simulink library "lib_env"  (Simulink 7.7)
settings: Solver=ode45  StartTime=0.0  StopTime=10.0  RelTol=1e-3
undefined symbols (not defined in the file): ADSW, area, arm, CD, CGP, CR, Earth, earth_radius, ele, GE, GGSW, GPperturbationSW, I, J2, jd, pSR, q_ini, rem_mag, rem_magSW, SGP, SRPSW, TOLERANCE, UT1_UTC, w_ini, wE, WGS84
libraries: lib_util x20, aerolibutil x13, lib_env x10, lib_orbittrance x9, aerolibtransform2 x6, lib_astrodynamics x5, aerolibatmos2 x1, vrlib x1, aerolibgravity2 x1
(part 2 of 2)

== matlab function IGRF11/IGRF11 ==
  data: fyears input double; B output double; alt input double; nlat input double; elong input double
function B=fnc(fyears,alt,nlat,elong)
%****************************************************
%  Direct conversion of igrf11_f to MATLAB
%  USAGE:   [B]=igrf11syn(fyears,alt,nlat,elong) 
% 
%  INPUT:   fyears = date in fractional years e.g. 1909.5 
%           alt    = altitude in                       (km)
%           nlat   = latiude positive north            (deg)
%           elong  = longitude positive east           (deg)
% OUTPUT:
%                B = [B_North; B_East; B_Up]           (nano Teslas)   ←間違い
%                B = [B_North; B_East; B_Down]         (nano Teslas)
% 2011/09/15 Update
% プログラムはNEDなのに、ここの表記がNEUになっていたのでNEDに変更
% この北極付近でプログラムの出力の第三成分は正の値になっていたことにより発覚
% (地磁気は北極がS極で、南極がN極なので北極付近では磁場ベクトルが地心方向を向く。
%  つまりDown方向を向く)
% ちなみにIGRF公式のc言語のプログラムにはNEDと書いてあった。

%  Conversion written by
%  Charles L. Rino
%  Rino Consulting
%  September 27 2010/October 3 2010 
%  crino@mindspring.com
%
%  CHANGES
%  date replaced by fyears
%  colat replaced by nlat
%  isv and itype preset to 0 and 1, respectively
%  output changed from [x,y,z,f] to non-redundant vector B=[x; y; z];
%The following text is from the fortran comment lines:
%
%     This is a program for synthesising geomagnetic field values from the 
%     International Geomagnetic Reference Field series of models as agreed
%     in December 2009 by IAGA Working Group V-MOD. 
%     It is the 11th generation IGRF, ie the 10th revision. 
%     The main-field models for 1900.0, 1905.0,..1940.0 and 2010.0 are 
%     non-definitive, those for 1945.0, 1950.0,...2005.0 are definitive and
%     the secular-variation model for 2010.0 to 2015.0 is non-definitive.
%
%     Main-field models are to degree and order 10 (ie 120 coefficients)
%     for 1900.0-1995.0 and to 13 (ie 195 coefficients) for 2000.0 onwards. 
%     The predictive secular-variation model is to degree and order 8 (ie 80
%     coefficients).
%
%     Options include values at different locations at different
%     times (spot), values at same location at one year intervals
%     (time series), grid of values at one time (grid); geodetic or
%     geocentric coordinates, latitude & longitude entered as decimal
%     degrees or degrees & minutes (not in grid), choice of main field 
%     or secular variation or both (grid only).
% Recent history of code:
%     Aug 2003: 
%     Adapted from 8th generation version to include new maximum degree for
%     main-field models for 2000.0 and onwards and use WGS84 spheroid instead
%     of International Astronomical Union 1966 spheroid as recommended by IAGA
%     in July 2003. Reference radius remains as 6371.2 km - it is NOT the mean
%     radius (= 6371.0 km) but 6371.2 km is what is used in determining the
%     coefficients. 
%     Dec 2004: 
%     Adapted for 10th generation
%     Jul 2005: 
%     1995.0 coefficients as published in igrf9coeffs.xls and igrf10coeffs.xls
%     now used in code - (Kimmo Korhonen spotted 1 nT difference in 11 coefficients)
%     Dec 2009:
%     Adapted for 11th generation
%
%   INPUT
%     isv   = 0 if main-field values are required
%     isv   = 1 if secular variation values are required
%     date  = year A.D. Must be greater than or equal to 1900.0 and
%             less than or equal to 2015.0. Warning message is given
%             for dates greater than 2010.0. Must be double precision.
%     itype = 1 if geodetic (spheroid)
%     itype = 2 if geocentric (sphere)
%     alt   = height in km above sea level if itype = 1
%           = distance from centre of Earth in km if itype = 2 (>3485 km)
%     colat = colatitude (0-180)
%     elong = east-longitude (0-360)
%     alt, colat and elong must be double precision.
%   OUTPUT
%     x     = north component (nT) if isv = 0, nT/year if isv = 1
%     y     = east component (nT) if isv = 0, nT/year if isv = 1
%     z     = vertical component (nT) if isv = 0, nT/year if isv = 1
%     f     = total intensity (nT) if isv = 0, rubbish if isv = 1
%     B     = [x; y; z]
%
%     To get the other geomagnetic elements (D, I, H and secular
%     variations dD, dH, dI and dF) use routines ptoc and ptocsv.
%
%     Adapted from 8th generation version to include new maximum degree for
%     main-field models for 2000.0 and onwards and use WGS84 spheroid instead
%     of International Astronomical Union 1966 spheroid as recommended by IAGA
%     in July 2003. Reference radius remains as 6371.2 km - it is NOT the mean
%     radius (= 6371.0 km) but 6371.2 km is what is used in determining the
%     coefficients. Adaptation by Susan Macmillan, August 2003 (for
%     9th generation) and December 2004.
%     1995.0 coefficients as published in igrf9coeffs.xls and igrf10coeffs.xls
%     used - (Kimmo Korhonen spotted 1 nT difference in 11 coefficients)
%     Susan Macmillan July 2005
%************************************************************************************
%global gh
gh = [-31543,-2298,5922,-677,2905,-1061,924,1121,1022,-1469,-330,1256,3,572,523,876,628,195,660,-69,-361,-210,134,-75,-184,328,-210,264,53,5,-33,-86,-124,-16,3,63,61,-9,-11,83,-217,2,-58,-35,59,36,-90,-69,70,-55,-45,0,-13,34,-10,-41,-1,-21,28,18,-12,6,-22,11,8,8,-4,-14,-9,7,1,-13,2,5,-9,16,5,-5,8,-18,8,10,-20,1,14,-11,5,12,-3,1,-2,-2,8,2,10,-1,-2,-1,2,-3,-4,2,2,1,-5,2,-2,6,6,-4,4,0,0,-2,2,4,2,0,0,-6,-31464,-2298,5909,-728,2928,-1086,1041,1065,1037,-1494,-357,1239,34,635,480,880,643,203,653,-77,-380,-201,146,-65,-192,328,-193,259,56,-1,-32,-93,-125,-26,11,62,60,-7,-11,86,-221,4,-57,-32,57,32,-92,-67,70,-54,-46,0,-14,33,-11,-41,0,-20,28,18,-12,6,-22,11,8,8,-4,-15,-9,7,1,-13,2,5,-8,16,5,-5,8,-18,8,10,-20,1,14,-11,5,12,-3,1,-2,-2,8,2,10,0,-2,-1,2,-3,-4,2,2,1,-5,2,-2,6,6,-4,4,0,0,-2,2,4,2,0,0,-6,-31354,-2297,5898,-769,2948,-1128,1176,1000,1058,-1524,-389,1223,62,705,425,884,660,211,644,-90,-400,-189,160,-55,-201,327,-172,253,57,-9,-33,-102,-126,-38,21,62,58,-5,-11,89,-224,5,-54,-29,54,28,-95,-65,71,-54,-47,1,-14,32,-12,-40,1,-19,28,18,-13,6,-22,11,8,8,-4,-15,-9,6,1,-13,2,5,-8,16,5,-5,8,-18,8,10,-20,1,14,-11,5,12,-3,1,-2,-2,8,2,10,0,-2,-1,2,-3,-4,2,2,1,-5,2,-2,6,6,-4,4,0,0,-2,2,4,2,0,0,-6,-31212,-2306,5875,-802,2956,-1191,1309,917,1084,-1559,-421,1212,84,778,360,887,678,218,631,-109,-416,-173,178,-51,-211,327,-148,245,58,-16,-34,-111,-126,-51,32,61,57,-2,-10,93,-228,8,-51,-26,49,23,-98,-62,72,-54,-48,2,-14,31,-12,-38,2,-18,28,19,-15,6,-22,11,8,8,-4,-15,-9,6,2,-13,3,5,-8,16,6,-5,8,-18,8,10,-20,1,14,-11,5,12,-3,1,-2,-2,8,2,10,0,-2,-1,2,-3,-4,2,2,1,-5,2,-2,6,6,-4,4,0,0,-2,1,4,2,0,0,-6,-31060,-2317,5845,-839,2959,-1259,1407,823,1111,-1600,-445,1205,103,839,293,889,695,220,616,-134,-424,-153,199,-57,-221,326,-122,236,58,-23,-38,-119,-125,-62,43,61,55,0,-10,96,-233,11,-46,-22,44,18,-101,-57,73,-54,-49,2,-14,29,-13,-37,4,-16,28,19,-16,6,-22,11,7,8,-3,-15,-9,6,2,-14,4,5,-7,17,6,-5,8,-19,8,10,-20,1,14,-11,5,12,-3,1,-2,-2,9,2,10,0,-2,-1,2,-3,-4,2,2,1,-5,2,-2,6,6,-4,4,0,0,-2,1,4,3,0,0,-6,-30926,-2318,5817,-893,2969,-1334,1471,728,1140,-1645,-462,1202,119,881,229,891,711,216,601,-163,-426,-130,217,-70,-230,326,-96,226,58,-28,-44,-125,-122,-69,51,61,54,3,-9,99,-238,14,-40,-18,39,13,-103,-52,73,-54,-50,3,-14,27,-14,-35,5,-14,29,19,-17,6,-21,11,7,8,-3,-15,-9,6,2,-14,4,5,-7,17,7,-5,8,-19,8,10,-20,1,14,-11,5,12,-3,1,-2,-2,9,2,10,0,-2,-1,2,-3,-4,2,2,1,-5,2,-2,6,6,-4,4,0,0,-2,1,4,3,0,0,-6,-30805,-2316,5808,-951,2980,-1424,1517,644,1172,-1692,-480,1205,133,907,166,896,727,205,584,-195,-422,-109,234,-90,-237,327,-72,218,60,-32,-53,-131,-118,-74,58,60,53,4,-9,102,-242,19,-32,-16,32,8,-104,-46,74,-54,-51,4,-15,25,-14,-34,6,-12,29,18,-18,6,-20,11,7,8,-3,-15,-9,5,2,-14,5,5,-6,18,8,-5,8,-19,8,10,-20,1,14,-12,5,12,-3,1,-2,-2,9,3,10,0,-2,-2,2,-3,-4,2,2,1,-5,2,-2,6,6,-4,4,0,0,-2,1,4,3,0,0,-6,-30715,-2306,5812,-1018,2984,-1520,1550,586,1206,-1740,-494,1215,146,918,101,903,744,188,565,-226,-415,-90,249,-114,-241,329,-51,211,64,-33,-64,-136,-115,-76,64,59,53,4,-8,104,-246,25,-25,-15,25,4,-106,-40,74,-53,-52,4,-17,23,-14,-33,7,-11,29,18,-19,6,-19,11,7,8,-3,-15,-9,5,1,-15,6,5,-6,18,8,-5,7,-19,8,10,-20,1,15,-12,5,11,-3,1,-3,-2,9,3,11,0,-2,-2,2,-3,-4,2,2,1,-5,2,-2,6,6,-4,4,0,0,-1,2,4,3,0,0,-6,-30654,-2292,5821,-1106,2981,-1614,1566,528,1240,-1790,-499,1232,163,916,43,914,762,169,550,-252,-405,-72,265,-141,-241,334,-33,208,71,-33,-75,-141,-113,-76,69,57,54,4,-7,105,-249,33,-18,-15,18,0,-107,-33,74,-53,-52,4,-18,20,-14,-31,7,-9,29,17,-20,5,-19,11,7,8,-3,-14,-10,5,1,-15,6,5,-5,19,9,-5,7,-19,8,10,-21,1,15,-12,5,11,-3,1,-3,-2,9,3,11,1,-2,-2,2,-3,-4,2,2,1,-5,2,-2,6,6,-4,4,0,0,-1,2,4,3,0,0,-6,-30594,-2285,5810,-1244,2990,-1702,1578,477,1282,-1834,-499,1255,186,913,-11,944,776,144,544,-276,-421,-55,304,-178,-253,346,-12,194,95,-20,-67,-142,-119,-82,82,59,57,6,6,100,-246,16,-25,-9,21,-16,-104,-39,70,-40,-45,0,-18,0,2,-29,6,-10,28,15,-17,29,-22,13,7,12,-8,-21,-5,-12,9,-7,7,2,-10,18,7,3,2,-11,5,-21,-27,1,17,-11,29,3,-9,16,4,-3,9,-4,6,-3,1,-4,8,-3,11,5,1,1,2,-20,-5,-1,-1,-6,8,6,-1,-4,-3,-2,5,0,-2,-2,-30554,-2250,5815,-1341,2998,-1810,1576,381,1297,-1889,-476,1274,206,896,-46,954,792,136,528,-278,-408,-37,303,-210,-240,349,3,211,103,-20,-87,-147,-122,-76,80,54,57,-1,4,99,-247,33,-16,-12,12,-12,-105,-30,65,-55,-35,2,-17,1,0,-40,10,-7,36,5,-18,19,-16,22,15,5,-4,-22,-1,0,11,-21,15,-8,-13,17,5,-4,-1,-17,3,-7,-24,-1,19,-25,12,10,2,5,2,-5,8,-2,8,3,-11,8,-7,-8,4,13,-1,-2,13,-10,-4,2,4,-3,12,6,3,-3,2,6,10,11,3,8,-30500,-2215,5820,-1440,3003,-1898,1581,291,1302,-1944,-462,1288,216,882,-83,958,796,133,510,-274,-397,-23,290,-230,-229,360,15,230,110,-23,-98,-152,-121,-69,78,47,57,-9,3,96,-247,48,-8,-16,7,-12,-107,-24,65,-56,-50,2,-24,10,-4,-32,8,-11,28,9,-20,18,-18,11,9,10,-6,-15,-14,5,6,-23,10,3,-7,23,6,-4,9,-13,4,9,-11,-4,12,-5,7,2,6,4,-2,1,10,2,7,2,-6,5,5,-3,-5,-4,-1,0,2,-8,-3,-2,7,-4,4,1,-2,-3,6,7,-2,-1,0,-3,-30421,-2169,5791,-1555,3002,-1967,1590,206,1302,-1992,-414,1289,224,878,-130,957,800,135,504,-278,-394,3,269,-255,-222,362,16,242,125,-26,-117,-156,-114,-63,81,46,58,-10,1,99,-237,60,-1,-20,-2,-11,-113,-17,67,-56,-55,5,-28,15,-6,-32,7,-7,23,17,-18,8,-17,15,6,11,-4,-14,-11,7,2,-18,10,4,-5,23,10,1,8,-20,4,6,-18,0,12,-9,2,1,0,4,-3,-1,9,-2,8,3,0,-1,5,1,-3,4,4,1,0,0,-1,2,4,-5,6,1,1,-1,-1,6,2,0,0,-7,-30334,-2119,5776,-1662,2997,-2016,1594,114,1297,-2038,-404,1292,240,856,-165,957,804,148,479,-269,-390,13,252,-269,-219,358,19,254,128,-31,-126,-157,-97,-62,81,45,61,-11,8,100,-228,68,4,-32,1,-8,-111,-7,75,-57,-61,4,-27,13,-2,-26,6,-6,26,13,-23,1,-12,13,5,7,-4,-12,-14,9,0,-16,8,4,-1,24,11,-3,4,-17,8,10,-22,2,15,-13,7,10,-4,-1,-5,-1,10,5,10,1,-4,-2,1,-2,-3,2,2,1,-5,2,-2,6,4,-4,4,0,0,-2,2,3,2,0,0,-6,-30220,-2068,5737,-1781,3000,-2047,1611,25,1287,-2091,-366,1278,251,838,-196,952,800,167,461,-266,-395,26,234,-279,-216,359,26,262,139,-42,-139,-160,-91,-56,83,43,64,-12,15,100,-212,72,2,-37,3,-6,-112,1,72,-57,-70,1,-27,14,-4,-22,8,-2,23,13,-23,-2,-11,14,6,7,-2,-15,-13,6,-3,-17,5,6,0,21,11,-6,3,-16,8,10,-21,2,16,-12,6,10,-4,-1,-5,0,10,3,11,1,-2,-1,1,-3,-3,1,2,1,-5,3,-1,4,6,-4,4,0,1,-1,0,3,3,1,-1,-4,-30100,-2013,5675,-1902,3010,-2067,1632,-68,1276,-2144,-333,1260,262,830,-223,946,791,191,438,-265,-405,39,216,-288,-218,356,31,264,148,-59,-152,-159,-83,-49,88,45,66,-13,28,99,-198,75,1,-41,6,-4,-111,11,71,-56,-77,1,-26,16,-5,-14,10,0,22,12,-23,-5,-12,14,6,6,-1,-16,-12,4,-8,-19,4,6,0,18,10,-10,1,-17,7,10,-21,2,16,-12,7,10,-4,-1,-5,-1,10,4,11,1,-3,-2,1,-3,-3,1,2,1,-5,3,-2,4,5,-4,4,-1,1,-1,0,3,3,1,-1,-5,-29992,-1956,5604,-1997,3027,-2129,1663,-200,1281,-2180,-336,1251,271,833,-252,938,782,212,398,-257,-419,53,199,-297,-218,357,46,261,150,-74,-151,-162,-78,-48,92,48,66,-15,42,93,-192,71,4,-43,14,-2,-108,17,72,-59,-82,2,-27,21,-5,-12,16,1,18,11,-23,-2,-10,18,6,7,0,-18,-11,4,-7,-22,4,9,3,16,6,-13,-1,-15,5,10,-21,1,16,-12,9,9,-5,-3,-6,-1,9,7,10,2,-6,-5,2,-4,-4,1,2,0,-5,3,-2,6,5,-4,3,0,1,-1,2,4,3,0,0,-6,-29873,-1905,5500,-2072,3044,-2197,1687,-306,1296,-2208,-310,1247,284,829,-297,936,780,232,361,-249,-424,69,170,-297,-214,355,47,253,150,-93,-154,-164,-75,-46,95,53,65,-16,51,88,-185,69,4,-48,16,-1,-102,21,74,-62,-83,3,-27,24,-2,-6,20,4,17,10,-23,0,-7,21,6,8,0,-19,-11,5,-9,-23,4,11,4,14,4,-15,-4,-11,5,10,-21,1,15,-12,9,9,-6,-3,-6,-1,9,7,9,1,-7,-5,2,-4,-4,1,3,0,-5,3,-2,6,5,-4,3,0,1,-1,2,4,3,0,0,-6,-29775,-1848,5406,-2131,3059,-2279,1686,-373,1314,-2239,-284,1248,293,802,-352,939,780,247,325,-240,-423,84,141,-299,-214,353,46,245,154,-109,-153,-165,-69,-36,97,61,65,-16,59,82,-178,69,3,-52,18,1,-96,24,77,-64,-80,2,-26,26,0,-1,21,5,17,9,-23,0,-4,23,5,10,-1,-19,-10,6,-12,-22,3,12,4,12,2,-16,-6,-10,4,9,-20,1,15,-12,11,9,-7,-4,-7,-2,9,7,8,1,-7,-6,2,-3,-4,2,2,1,-5,3,-2,6,4,-4,3,0,1,-2,3,3,3,-1,0,-6,-29692,-1784,5306,-2200,3070,-2366,1681,-413,1335,-2267,-262,1249,302,759,-427,940,780,262,290,-236,-418,97,122,-306,-214,352,46,235,165,-118,-143,-166,-55,-17,107,68,67,-17,68,72,-170,67,-1,-58,19,1,-93,36,77,-72,-69,1,-25,28,4,5,24,4,17,8,-24,-2,-6,25,6,11,-6,-21,-9,8,-14,-23,9,15,6,11,-5,-16,-7,-4,4,9,-20,3,15,-10,12,8,-6,-8,-8,-1,8,10,5,-2,-8,-8,3,-3,-6,1,2,0,-4,4,-1,5,4,-5,2,-1,2,-2,5,1,1,-2,0,-7,0,0,0,0,0,0,0,0,0,0,0,0,0,0,0,0,0,0,0,0,0,0,0,0,0,0,0,0,0,0,0,0,0,0,0,0,0,0,0,0,0,0,0,0,0,0,0,0,0,0,0,0,0,0,0,0,0,0,0,0,0,0,0,0,0,0,0,0,0,0,0,0,0,0,0,-29619.4000000000,-1728.20000000000,5186.10000000000,-2267.70000000000,3068.40000000000,-2481.60000000000,1670.90000000000,-458,1339.60000000000,-2288,-227.600000000000,1252.10000000000,293.400000000000,714.500000000000,-491.100000000000,932.300000000000,786.800000000000,272.600000000000,250,-231.900000000000,-403,119.800000000000,111.300000000000,-303.800000000000,-218.800000000000,351.400000000000,43.8000000000000,222.300000000000,171.900000000000,-130.400000000000,-133.100000000000,-168.600000000000,-39.3000000000000,-12.9000000000000,106.300000000000,72.3000000000000,68.2000000000000,-17.4000000000000,74.2000000000000,63.7000000000000,-160.900000000000,65.1000000000000,-5.90000000000000,-61.2000000000000,16.9000000000000,0.700000000000000,-90.4000000000000,43.8000000000000,79,-74,-64.6000000000000,0,-24.2000000000000,33.3000000000000,6.20000000000000,9.10000000000000,24,6.90000000000000,14.8000000000000,7.30000000000000,-25.4000000000000,-1.20000000000000,-5.80000000000000,24.4000000000000,6.60000000000000,11.9000000000000,-9.20000000000000,-21.5000000000000,-7.90000000000000,8.50000000000000,-16.6000000000000,-21.5000000000000,9.10000000000000,15.5000000000000,7,8.90000000000000,-7.90000000000000,-14.9000000000000,-7,-2.10000000000000,5,9.40000000000000,-19.7000000000000,3,13.4000000000000,-8.40000000000000,12.5000000000000,6.30000000000000,-6.20000000000000,-8.90000000000000,-8.40000000000000,-1.50000000000000,8.40000000000000,9.30000000000000,3.80000000000000,-4.30000000000000,-8.20000000000000,-8.20000000000000,4.80000000000000,-2.60000000000000,-6,1.70000000000000,1.70000000000000,0,-3.10000000000000,4,-0.500000000000000,4.90000000000000,3.70000000000000,-5.90000000000000,1,-1.20000000000000,2,-2.90000000000000,4.20000000000000,0.200000000000000,0.300000000000000,-2.20000000000000,-1.10000000000000,-7.40000000000000,2.70000000000000,-1.70000000000000,0.100000000000000,-1.90000000000000,1.30000000000000,1.50000000000000,-0.900000000000000,-0.100000000000000,-2.60000000000000,0.100000000000000,0.900000000000000,-0.700000000000000,-0.700000000000000,0.700000000000000,-2.80000000000000,1.70000000000000,-0.900000000000000,0.100000000000000,-1.20000000000000,1.20000000000000,-1.90000000000000,4,-0.900000000000000,-2.20000000000000,-0.300000000000000,-0.400000000000000,0.200000000000000,0.300000000000000,0.900000000000000,2.50000000000000,-0.200000000000000,-2.60000000000000,0.900000000000000,0.700000000000000,-0.500000000000000,0.300000000000000,0.300000000000000,0,-0.300000000000000,0,-0.400000000000000,0.300000000000000,-0.100000000000000,-0.900000000000000,-0.200000000000000,-0.400000000000000,-0.400000000000000,0.800000000000000,-0.200000000000000,-0.900000000000000,-0.900000000000000,0.300000000000000,0.200000000000000,0.100000000000000,1.80000000000000,-0.400000000000000,-0.400000000000000,1.30000000000000,-1,-0.400000000000000,-0.100000000000000,0.700000000000000,0.700000000000000,-0.400000000000000,0.300000000000000,0.300000000000000,0.600000000000000,-0.100000000000000,0.300000000000000,0.400000000000000,-0.200000000000000,0,-0.500000000000000,0.100000000000000,-0.900000000000000,-29554.6300000000,-1669.05000000000,5077.99000000000,-2337.24000000000,3047.69000000000,-2594.50000000000,1657.76000000000,-515.430000000000,1336.30000000000,-2305.83000000000,-198.860000000000,1246.39000000000,269.720000000000,672.510000000000,-524.720000000000,920.550000000000,797.960000000000,282.070000000000,210.650000000000,-225.230000000000,-379.860000000000,145.150000000000,100,-305.360000000000,-227,354.410000000000,42.7200000000000,208.950000000000,180.250000000000,-136.540000000000,-123.450000000000,-168.050000000000,-19.5700000000000,-13.5500000000000,103.850000000000,73.6000000000000,69.5600000000000,-20.3300000000000,76.7400000000000,54.7500000000000,-151.340000000000,63.6300000000000,-14.5800000000000,-63.5300000000000,14.5800000000000,0.240000000000000,-86.3600000000000,50.9400000000000,79.8800000000000,-74.4600000000000,-61.1400000000000,-1.65000000000000,-22.5700000000000,38.7300000000000,6.82000000000000,12.3000000000000,25.3500000000000,9.37000000000000,10.9300000000000,5.42000000000000,-26.3200000000000,1.94000000000000,-4.64000000000000,24.8000000000000,7.62000000000000,11.2000000000000,-11.7300000000000,-20.8800000000000,-6.88000000000000,9.83000000000000,-18.1100000000000,-19.7100000000000,10.1700000000000,16.2200000000000,9.36000000000000,7.61000000000000,-11.2500000000000,-12.7600000000000,-4.87000000000000,-0.0600000000000000,5.58000000000000,9.76000000000000,-20.1100000000000,3.58000000000000,12.6900000000000,-6.94000000000000,12.6700000000000,5.01000000000000,-6.72000000000000,-10.7600000000000,-8.16000000000000,-1.25000000000000,8.10000000000000,8.76000000000000,2.92000000000000,-6.66000000000000,-7.73000000000000,-9.22000000000000,6.01000000000000,-2.17000000000000,-6.12000000000000,2.19000000000000,1.42000000000000,0.100000000000000,-2.35000000000000,4.46000000000000,-0.150000000000000,4.76000000000000,3.06000000000000,-6.58000000000000,0.290000000000000,-1.01000000000000,2.06000000000000,-3.47000000000000,3.77000000000000,-0.860000000000000,-0.210000000000000,-2.31000000000000,-2.09000000000000,-7.93000000000000,2.95000000000000,-1.60000000000000,0.260000000000000,-1.88000000000000,1.44000000000000,1.44000000000000,-0.770000000000000,-0.310000000000000,-2.27000000000000,0.290000000000000,0.900000000000000,-0.790000000000000,-0.580000000000000,0.530000000000000,-2.69000000000000,1.80000000000000,-1.08000000000000,0.160000000000000,-1.58000000000000,0.960000000000000,-1.90000000000000,3.99000000000000,-1.39000000000000,-2.15000000000000,-0.290000000000000,-0.550000000000000,0.210000000000000,0.230000000000000,0.890000000000000,2.38000000000000,-0.380000000000000,-2.63000000000000,0.960000000000000,0.610000000000000,-0.300000000000000,0.400000000000000,0.460000000000000,0.0100000000000000,-0.350000000000000,0.0200000000000000,-0.360000000000000,0.280000000000000,0.0800000000000000,-0.870000000000000,-0.490000000000000,-0.340000000000000,-0.0800000000000000,0.880000000000000,-0.160000000000000,-0.880000000000000,-0.760000000000000,0.300000000000000,0.330000000000000,0.280000000000000,1.72000000000000,-0.430000000000000,-0.540000000000000,1.18000000000000,-1.07000000000000,-0.370000000000000,-0.0400000000000000,0.750000000000000,0.630000000000000,-0.260000000000000,0.210000000000000,0.350000000000000,0.530000000000000,-0.0500000000000000,0.380000000000000,0.410000000000000,-0.220000000000000,-0.100000000000000,-0.570000000000000,-0.180000000000000,-0.820000000000000,-29496.5000000000,-1585.90000000000,4945.10000000000,-2396.60000000000,3026,-2707.70000000000,1668.60000000000,-575.400000000000,1339.70000000000,-2326.30000000000,-160.500000000000,1231.70000000000,251.700000000000,634.200000000000,-536.800000000000,912.600000000000,809,286.400000000000,166.600000000000,-211.200000000000,-357.100000000000,164.400000000000,89.7000000000000,-309.200000000000,-231.100000000000,357.200000000000,44.7000000000000,200.300000000000,188.900000000000,-141.200000000000,-118.100000000000,-163.100000000000,0.100000000000000,-7.70000000000000,100.900000000000,72.8000000000000,68.6000000000000,-20.8000000000000,76,44.2000000000000,-141.400000000000,61.5000000000000,-22.9000000000000,-66.3000000000000,13.1000000000000,3.10000000000000,-77.9000000000000,54.9000000000000,80.4000000000000,-75,-57.8000000000000,-4.70000000000000,-21.2000000000000,45.3000000000000,6.60000000000000,14,24.9000000000000,10.4000000000000,7,1.60000000000000,-27.7000000000000,4.90000000000000,-3.40000000000000,24.3000000000000,8.20000000000000,10.9000000000000,-14.5000000000000,-20,-5.70000000000000,11.9000000000000,-19.3000000000000,-17.4000000000000,11.6000000000000,16.7000000000000,10.9000000000000,7.10000000000000,-14.1000000000000,-10.8000000000000,-3.70000000000000,1.70000000000000,5.40000000000000,9.40000000000000,-20.5000000000000,3.40000000000000,11.6000000000000,-5.30000000000000,12.8000000000000,3.10000000000000,-7.20000000000000,-12.4000000000000,-7.40000000000000,-0.800000000000000,8,8.40000000000000,2.20000000000000,-8.40000000000000,-6.10000000000000,-10.1000000000000,7,-2,-6.30000000000000,2.80000000000000,0.900000000000000,-0.100000000000000,-1.10000000000000,4.70000000000000,-0.200000000000000,4.40000000000000,2.50000000000000,-7.20000000000000,-0.300000000000000,-1,2.20000000000000,-4,3.10000000000000,-2,-1,-2,-2.80000000000000,-8.30000000000000,3,-1.50000000000000,0.100000000000000,-2.10000000000000,1.70000000000000,1.60000000000000,-0.600000000000000,-0.500000000000000,-1.80000000000000,0.500000000000000,0.900000000000000,-0.800000000000000,-0.400000000000000,0.400000000000000,-2.50000000000000,1.80000000000000,-1.30000000000000,0.200000000000000,-2.10000000000000,0.800000000000000,-1.90000000000000,3.80000000000000,-1.80000000000000,-2.10000000000000,-0.200000000000000,-0.800000000000000,0.300000000000000,0.300000000000000,1,2.20000000000000,-0.700000000000000,-2.50000000000000,0.900000000000000,0.500000000000000,-0.100000000000000,0.600000000000000,0.500000000000000,0,-0.400000000000000,0.100000000000000,-0.400000000000000,0.300000000000000,0.200000000000000,-0.900000000000000,-0.800000000000000,-0.200000000000000,0,0.800000000000000,-0.200000000000000,-0.900000000000000,-0.800000000000000,0.300000000000000,0.300000000000000,0.400000000000000,1.70000000000000,-0.400000000000000,-0.600000000000000,1.10000000000000,-1.20000000000000,-0.300000000000000,-0.100000000000000,0.800000000000000,0.500000000000000,-0.200000000000000,0.100000000000000,0.400000000000000,0.500000000000000,0,0.400000000000000,0.400000000000000,-0.200000000000000,-0.300000000000000,-0.500000000000000,-0.300000000000000,-0.800000000000000,11.4000000000000,16.7000000000000,-28.8000000000000,-11.3000000000000,-3.90000000000000,-23,2.70000000000000,-12.9000000000000,1.30000000000000,-3.90000000000000,8.60000000000000,-2.90000000000000,-2.90000000000000,-8.10000000000000,-2.10000000000000,-1.40000000000000,2,0.400000000000000,-8.90000000000000,3.20000000000000,4.40000000000000,3.60000000000000,-2.30000000000000,-0.800000000000000,-0.500000000000000,0.500000000000000,0.500000000000000,-1.50000000000000,1.50000000000000,-0.700000000000000,0.900000000000000,1.30000000000000,3.70000000000000,1.40000000000000,-0.600000000000000,-0.300000000000000,-0.300000000000000,-0.100000000000000,-0.300000000000000,-2.10000000000000,1.90000000000000,-0.400000000000000,-1.60000000000000,-0.500000000000000,-0.200000000000000,0.800000000000000,1.80000000000000,0.500000000000000,0.200000000000000,-0.100000000000000,0.600000000000000,-0.600000000000000,0.300000000000000,1.40000000000000,-0.200000000000000,0.300000000000000,-0.100000000000000,0.100000000000000,-0.800000000000000,-0.800000000000000,-0.300000000000000,0.400000000000000,0.200000000000000,-0.100000000000000,0.100000000000000,0,-0.500000000000000,0.200000000000000,0.300000000000000,0.500000000000000,-0.300000000000000,0.400000000000000,0.300000000000000,0.100000000000000,0.200000000000000,-0.100000000000000,-0.500000000000000,0.400000000000000,0.200000000000000,0.400000000000000,0,0,0,0,0,0,0,0,0,0,0,0,0,0,0,0,0,0,0,0,0,0,0,0,0,0,0,0,0,0,0,0,0,0,0,0,0,0,0,0,0,0,0,0,0,0,0,0,0,0,0,0,0,0,0,0,0,0,0,0,0,0,0,0,0,0,0,0,0,0,0,0,0,0,0,0,0,0,0,0,0,0,0,0,0,0,0,0,0,0,0,0,0,0,0,0,0,0,0,0,0,0,0,0,0,0,0,0,0,0,0,0,0,0,0;];
%%%%%%%%%%%Variable Changes:
isv=0;
itype=1;
colat=90-nlat;
%****************************************************
cl=NaN*ones(1,13); 
sl=NaN*ones(1,13);  
x     = 0;
y     = 0;
z     = 0;
if fyears < 1900 || fyears > 2020
    error('Date >=1900 & <=2020')
end
%if fyears > 2015
%    warning('on',' This version of IGRF intended for use to only to 2015 \n')
%end
if fyears <2010
    t     = 0.2*(fyears - 1900.0);
    ll    = floor(t);
    one   = ll;
    t     = t - one;
    if fyears<1995.0 
        nmx   = 10;
        nc    = nmx*(nmx+2);
        ll    = nc*ll;
        kmx   = (nmx+1)*(nmx+2)/2;
    else %1995<=fyears<2010
        nmx   = 13;
        nc    = nmx*(nmx+2);
        ll    = floor(0.2*(fyears - 1995));
        ll    = 120*19 + nc*ll;
        kmx   = (nmx+1)*(nmx+2)/2;
    end
    tc  = 1-t;
    if isv==1
        tc = -0.2;
        t  = 0.2;
    end
else %>= 2010
    t=fyears-2010;
    tc =1;
    if isv==1
        t=1;
        tc=0;
    end
    ll    = 2865;
    nmx   = 13;
    nc    = nmx*(nmx+2);
    kmx   = (nmx+1)*(nmx+2)/2;
end

r     = alt;
one   = colat*0.017453292;
ct    = cos(one);
st    = sin(one);
one   = elong*0.017453292;
cl(1) = cos(one);
sl(1) = sin(one);
cd    = 1.0;
sd    = 0.0;
l     = 1;
m     = 1;
n     = 0;

if itype==1  %Skip if itype==2
    %   Conversion from geodetic to geocentric coordinates (using the WGS84 spheroid)
    a2    = 40680631.6;
    b2    = 40408296.0;
    one   = a2*st*st;
    two   = b2*ct*ct;
    three = one + two;
    rho   = sqrt(three);
    r     = sqrt(alt*(alt + 2.0*rho) + (a2*one + b2*two)/three);
    cd    = (alt + rho)/r;
    sd    = (a2 - b2)/rho*ct*st/r;
    one   = ct;
    ct    = ct*cd -  st*sd;
    st    = st*cd + one*sd;
end
ratio = 6371.2/r;  
rr    = ratio*ratio;
p=NaN*ones(1,kmx);
q=NaN*ones(1,kmx);

fn = 0.0;
gn = 0.0;

%     computation of Schmidt quasi-normal coefficients p and x(=q)
p(1)  = 1.0;
p(3)  = st;
q(1)  = 0.0;
q(3)  =  ct;
for k=2:kmx
    if n<m
        m     = 0;
        n     = n + 1;
        rr    = rr*ratio;
        fn    = n;
        gn    = n - 1;
    end
    fm    = m;
    if m==n && k~=3
        one   = sqrt(1.0 - 0.5/fm);
        j     = k - n - 1;
        p(k)  = one*st*p(j);
        q(k)  = one*(st*q(j) + ct*p(j));
        cl(m) = cl(m-1)*cl(1) - sl(m-1)*sl(1);
        sl(m) = sl(m-1)*cl(1) + cl(m-1)*sl(1);
    end
    if m~=n && k~=3
        gmm    = m*m;
        one   = sqrt(fn*fn - gmm);
        two   = sqrt(gn*gn - gmm)/one;
        three = (fn + gn)/one;
        i     = k - n;
        j     = i - n + 1;
        p(k)  = three*ct*p(i) - two*p(j);
        q(k)  = three*(ct*q(i) - st*p(i)) - two*q(j);
    end
    %Synthesis of x, y, and z
    lm    = ll + l;
    one   = (tc*gh(lm) + t*gh(lm+nc))*rr;
    %DEBUG 
    %[nyear,ncoef]=decode_coeff_pointer(lm);
    %fprintf('nyear %6i %5i %5i \n',lm,nyear,ncoef); 
    if m~=0
        two   = (tc*gh(lm+1) + t*gh(lm+nc+1))*rr;
        three = one*cl(m) + two*sl(m);
        x     = x + three*q(k);
        z     = z - (fn + 1.0)*three*p(k);
        if st~=0
            y     = y + (one*sl(m) - two*cl(m))*fm*p(k)/st;
        else
            y     = y + (one*sl(m) - two*cl(m))*q(k)*ct;
        end
        l     = l + 2;
    else
        x     = x + one*q(k);
        z     = z - (fn + 1.0)*one*p(k);
        l     = l + 1;
    end
    m     = m + 1;
end %k loop

%     conversion to coordinate system specified by itype
one   = x;
x     = x*cd +   z*sd;
z     = z*cd - one*sd;
B     =[x; y; z];
%f     = sqrt(x*x + y*y + z*z);
return

== matlab function OEtoSATPOS/sat_IJK ==
  data: ele input double; th input double; r input double; pos output double; R input double; v output double
function [pos,v]  = sat_pos(ele,th,r,R)
%#codegen
%calculate sat pos and vel
GE=3.986004415*(10^5); % km^3/s^2

a=ele(1);
e=ele(2); 
W=ele(4);
i=ele(3);
ww=ele(5);

u = ww + th;
p = a * (1.0 -e * e);
h = sqrt(GE * p);

cu = cos(u);
su = sin(u);
ci = cos(i);
si = sin(i);
cW = cos(W);
sW = sin(W);

x=r*(cu*cW-su*ci*sW);
y=r*(cu*sW+su*ci*cW);
z=r*su*si;

pos=[x;y;z];

r_dot=h/a/(1-e*e)*e*sin(th);
f_dot=h/r/r;
%   vx = r_dot*R(1,1)+r*f_dot*R(1,2); %/* vx[km/s] */
%   vy = r_dot*R(2,1)+r*f_dot*R(2,2); %/* vy[km/s] */
%   vz = r_dot*R(3,1)+r*f_dot*R(3,2); %/* vz[km/s] */
vx = r_dot*(cW*cu-sW*su*ci)+r*f_dot*(-cW*su-sW*cu*ci); %/* vx[km/s] */
vy = r_dot*(sW*cu+cW*su*ci)+r*f_dot*(-sW*su+cW*cu*ci); %/* vy[km/s] */
vz = r_dot*(su*si)+r*f_dot*(cu*si); %/* vz[km/s] */
v=[vx;vy;vz];

== matlab function dipole geomagnetic model ==
  data: rsat_e input double; B output double
function B = fcn(rsat_e)
%#codegen

M = 7.789e+15; % nT km^3
delta = 79.530 / 180.0 * pi;
alpha = 288.348 / 180.0 * pi;

cd = cos(delta);
sd = sin(delta);
ca = cos(alpha);
sa = sin(alpha);

norm_rsat_e = norm(rsat_e);
r = rsat_e / norm_rsat_e;

d = -[cd * ca; cd * sa; sd];



norm_rsat_e3 = norm_rsat_e * norm_rsat_e * norm_rsat_e;
B = M / norm_rsat_e3 * (3.0 * (d' * r) * r - d);

== matlab function Atmosdence/MATLAB Function ==
  data: year input double; dy output double; month input double; day input double; hour input double; minute input double; second input double
function dy = DOY(year, month, day, hour, minute, second)
%#codegen

days_in_prev_months = [0 31 59 90 120 151 181 212 243 273 304 334]';

% Day in given month.
dy = days_in_prev_months(month) ...                % days in prev. months
   + (isleapyear(year) & (month > 2)) ...          % leap day
   + day ...                                       % day in month
   + (second + 60 * minute + 3600 * hour) / 86400; % part of day

function t = isleapyear(year)
	t = (~rem(year, 4) & rem(year, 100)) | ~rem(year, 400);

== matlab function nonsphericaleffect/m2km ==
  data: u input double; y output double
function y = fcn(u)
%#codegen

y = 1/1000*u';

== matlab function AirDrag/calc_AD ==
  data: ro input double; AD_acc output double; area input double; r input double; ele input double; th input double; R input double; mass input double; AD_t output double

function  [AD_acc, AD_t] = AirDrag(ro,area,r,ele,th,R,mass)
%#codegen
    
 EARTH_ROTATION =6.30038809898489122118/24.0/3600.0; % rad/sec
 CD = 2.2; %(2~2.5)
 arm=0.05;%cm
 GE=3.986004415*(10^5); % km^3/s^2
  
 a=ele(1);
 e=ele(2);
 p = a * (1.0 -e * e);
 h = sqrt(GE * p);
 
    v1 = h * e * sin (th) / p;
    v2 = h / r - EARTH_ROTATION * r *R(3,2);
    v3 =         EARTH_ROTATION * r *R(3,1);
    
    ap = 0.5 * CD * area * ro * sqrt(v1^2+v2^2+v3^2); 
    
    AD_acc =(1000/mass)*[-ap * v1; -ap * v2; - ap * v3];
    AD_t=(1000^2)*arm*[-ap * v1; -ap * v2; - ap * v3];

== matlab function nonsphericaleffect/makeline ==
  data: u input double; y output double; v input double
function y = fcn(u,v)
%#codegen

y = [u',v];

== matlab function Non-spherical term ==
  data: phi input double; lam input double; pos input double; a output double; R input double

function a  = Gperturb(phi,lam,pos,R)
%#codegen
r=sqrt(pos(1)^2+pos(2)^2+pos(3)^2);
GE=3.986004415*(10^5); % km^3/s^2
Re=6378.1363; % km
J2=0.1082626925638815E-2;
C22=0.1574421758350994E-5;
S22=-0.9037666669616874E-6;

dU_dr=GE/r/r*J2*((Re/r)^2)*3/2*(3*sin(phi*pi/180)*sin(phi*pi/180)-1)...
    -GE/r/r*((Re/r)^2)*3*(3*cos(phi*pi/180)*cos(phi*pi/180)*(C22*cos(2*lam*pi/180)+S22*sin(2*lam*pi/180)));
dU_dp=-GE/r*J2*((Re/r)^2)*3*sin(phi*pi/180)*cos(phi*pi/180)...
    +GE/r*((Re/r)^2)*(-2*tan(phi*pi/180)*3*cos(phi*pi/180)*cos(phi*pi/180))*(C22*cos(2*lam*pi/180)+S22*sin(2*lam*pi/180));
dU_dl=GE/r*((Re/r)^2)*(3*cos(phi*pi/180)*cos(phi*pi/180))*(S22*cos(2*lam*pi/180)-C22*sin(2*lam*pi/180));

ar=dU_dr;
as=R(3,2)/cos(phi*pi/180)/r*dU_dp+R(3,3)/cos(phi*pi/180)/r/cos(phi*pi/180)*dU_dl;
aw=R(3,3)/cos(phi*pi/180)/r*dU_dp-R(3,2)/cos(phi*pi/180)/r/cos(phi*pi/180)*dU_dl;
%IJK<->RSW この項は一致
a=[ar,as,aw];

== matlab function pwr_generaton/solargeneration ==
  data: sun input double; padol output double; sun_flag input double; padol_flag input double; x_p output double; z_y_p output double; l_sun_out output double; cell_c input double; cell_o input double
function [padol,x_p,z_y_p,l_sun_out] =  fcn(sun,sun_flag,padol_flag,cell_c,cell_o)
%#codegen

if sun_flag == 0
    power=zeros(6,1);
    l_sun_out=zeros(6,1);
else
    sun=sun/norm(sun);
    %x
    f = [1; 0;  0];
    costheta = sun' * f;
        if costheta > 0
            plus_x=costheta;%acos(costheta);
            minus_x = 0;
        else
            plus_x= 0;
            minus_x =-costheta;% acos(-costheta);
        end

    %+y
    f = [0; 1; 0];
    costheta = sun' * f;
        if costheta > 0
            plus_y=costheta;%acos(costheta);
            minus_y = 0;
        else
            plus_y= 0;
            minus_y =-costheta ;%acos(-costheta);
        end
    
    %z
    f = [0; 0; 1];
    costheta = sun' * f;
    
       if costheta > 0
            plus_z=costheta;%acos(costheta);
            minus_z = 0;
       else
            plus_z= 0;
            minus_z =-costheta;% acos(-costheta);
        end
    l_sun_out = [minus_x;plus_x;minus_y;plus_y;minus_z;plus_z];
    
        if padol_flag == 0
            cell=cell_c;
        else
            cell=cell_o;
        end
        
    power = [cell(1) 0 0 0 0 0;...
             0 cell(2)  0 0 0 0;...
             0  0 cell(3) 0 0 0;...
             0  0 0 cell(4) 0 0;...
             0  0 0 0 cell(5) 0;...
             0  0 0 0 0 cell(6)]*l_sun_out;        
end

         if padol_flag == 0
             padol=power(5)+power(3)+power(4);
             x_p=power(1)+power(2);
             z_y_p=power(6);
         else
             padol=power(5);
             x_p=power(1)+power(2);
             z_y_p=power(3)+power(4)+power(6);            
         end

== matlab function SRP/srp ==
  data: jd input double; pos input double; SRP_acc output double; r input double; R input double; area input double; mass input double; SRP_t output double
function[SRP_acc, SRP_t]= srp(jd,pos,r,R,area,mass)
%#codegen
% rp:taiyou vec
	t = ( jd - 2451545.0 ) / 36525.0;
	
	M =DegtoRad(357.5256+35999.045*t);
	l =DegtoRad(282.94+M/pi*180.0+SecToDeg(6892)*sin(M)+SecToDeg(72)*sin(2*M)-(0.002652-SecToDeg(1250.09115*t)));
	rp =149619000-2499000*cos(M)-21000*cos(2*M);
    
epsilon=23.43929111*pi/180.0;
  sun=[ cos(l); cos(epsilon)*sin(l); sin(epsilon)*sin(l)];
  s=(pos')*sun;

arm=0.05;

  a =cos(l);
  b =cos(epsilon)*sin(l);
  g = sin(epsilon)*sin(l);
  
  SRP_CONST=1367/(3*10^8)*1000;
  KE_PER_AU=149597870.0;
  rp=rp/KE_PER_AU;

  if (s > 0 || sqrt (r * r - s * s) > 6378.1363)
  ap = 1.2 * SRP_CONST * (area/mass) /rp;% (rp * rp);%  Reflectivity = 1.2 (1~2)

  fr = -ap * (R(1,1) * a + R(2,1) * b + R(3,1) * g);
  fs = -ap * (R(1,2) * a + R(2,2) * b + R(3,2) * g);
  fw = -ap * (R(1,3) * a + R(2,3) * b + R(3,3) * g);
  else
      fr=0;fs=0;fw=0;
  end

  F=[fr;fs;fw];
  
  SRP_acc = F/1000;
  SRP_t =  F*mass*arm;
  
  function rad = DegtoRad(ang)
	ang = ang-floor(ang/360.0)*360.0;
	rad = ang*pi/180.0;
    
function deg=SecToDeg (ang)

	deg = ang/3600;

== matlab function pwrbudget_cal/Efficiency ==
  data: u input double; y output double
function y = fcn(u)
%#codegen
effeciency=0.8;
if u > 0
    y= effeciency*u;
else
    y=u;
end

== matlab function Sun_bodyeffect/sun_b_e ==
  data: lon input double; lat input double; rp input double; F output double; ele input double; r input double; R input double
function F = sun_body_eff(lon, lat, rp, ele,r,R)
%#codegen
% rp:taiyou vec

GS=1.327124*10^11;% km^3/s^2
%y=[cu, ci, cn, ce,su,si,sn,se]
e=ele(2);
ce=cos(e);%y(4);
se=sin(e);%y(8);

  a = cos (lat) * cos (lon);
  b = ce * cos (lat) * sin (lon) - se * sin (lat);
  g = se * cos (lat) * sin (lon) + ce * sin (lat);

  r1 = rp * a - r * R(1,1);
  r2 = rp * b - r * R(1,2);
  r3 = rp * g - r * R(1,3);

  r23 = sqrt (r1 * r1 + r2 * r2 + r3 * r3); 
  r23 = r23 * r23 * r23;

  ap = GS * (rp / r23 - 1.0/ (rp * rp));

  fr = ap * (R(1,1) * a + R(2,1) * b + R(3,1) * g) - GS * r / r23; 
  fs = ap * (R(1,2) * a + R(2,2) * b + R(3,2) * g);                
  fw = ap * (R(1,3) * a + R(2,3) * b + R(3,3) * g); 
  
  F=[fr;fs;fw];

== matlab function Moon_bodyeffect/moonbodyeffect ==
  data: lon input double; lat input double; rp input double; F output double; ele input double; r input double; R input double
function F = moon_body_eff(lon, lat,rp,  ele ,r,R)
%#codegen
% rp:taiyou vec

GM=4902.798882;% km^3/s^2
%y=[cu, ci, cn, ce,su,si,sn,se]
e=ele(2);
ce=cos(e);%y(4);
se=sin(e);%y(8);

  a = cos (lat) * cos (lon);
  b = ce * cos (lat) * sin (lon) - se * sin (lat);
  g = se * cos (lat) * sin (lon) + ce * sin (lat);

  r1 = rp * a - r * R(1,1);
  r2 = rp * b - r * R(1,2);
  r3 = rp * g - r * R(1,3);

  r23 = sqrt (r1 * r1 + r2 * r2 + r3 * r3); 
  r23 = r23 * r23 * r23;

  ap = GM * (rp / r23 - 1.0/ (rp * rp));

  fr = ap * (R(1,1) * a + R(2,1) * b + R(3,1) * g) - GM * r / r23; 
  fs = ap * (R(1,2) * a + R(2,2) * b + R(3,2) * g);                
  fw = ap * (R(1,3) * a + R(2,3) * b + R(3,3) * g); 
  
  F=[fr;fs;fw];

== matlab function Perturbation&Disturabance/MATLAB Function ==
  data: CGP input double; SGP input double; Re input double; phi input double; lam input double; r input double; i input double; u input double; a output double
function a = fcn(CGP, SGP, Re, phi, lam, r, i, u)
%#codegen

a = calcForce(CGP, SGP, Re, phi, lam, r, i, u);

== matlab function Sun_flag/srp ==
  data: jd input double; pos input double; flag output double; r input double
function flag = srp(jd,pos,r)
%#codegen
% rp:taiyou vec
  
	t = ( jd - 2451545.0 ) / 36525.0;
	
	M =DegtoRad(357.5256+35999.045*t);
	l =DegtoRad(282.94+M/pi*180.0+SecToDeg(6892)*sin(M)+SecToDeg(72)*sin(2*M)-(0.002652-SecToDeg(1250.09115*t)));

epsilon=23.43929111*pi/180.0;
  sun=[ cos(l); cos(epsilon)*sin(l); sin(epsilon)*sin(l)];
  s=(pos')*sun;
  if (s > 0 || sqrt (r * r - s * s) > 6378.1363)
      flag = 1;
  else
      flag = 0;
  end
  
  function rad = DegtoRad(ang)
	ang = ang-floor(ang/360.0)*360.0;
	rad = ang*pi/180.0;
        
function deg=SecToDeg (ang)

	deg = ang/3600;

== matlab function pwrbudget_cal/pwrload ==
  data: u input double; p output double
function p = pwrload(u)
%#codegen

p=0;

% 0: safe mode
% 1:only MOBC
% 2:only MOBC+AOBC
% 3:Sun pointing spin

if u==0
    p=5.9;
end
if u==1
    p=12.3;
end
if u==2
    p=18.7;
end
if u==3
    21.9;
end

== matlab function nrlmsise-00 simple/MATLAB Function ==
  data: UT input double; LST output double; lon input double
function LST = fcn(UT,lon)
%#codegen

LST = UT / 3600 + lon / 15;

== matlab function half angle separation of the earth/MATLAB Function ==
  data: h input double; ang output double; R input double
function ang = fcn(h, R)
%#codegen

ang = asin(R / (R + h));

== matlab function Environment&Dynamics/Air Drag/Air Drag ==
  data: rho input double; F output double; CD input double; A input double; v input double
function F = fcn(rho, CD, A, v)
%#codegen

% rho: atmospheric density[kg/m^3]
% A  : cross section of satellite[m^2]
% v  : satellite velocity[km/s]

norm_v = norm(v);

F = -0.5 * rho * CD * A * norm_v * v;
% kg / m^3 * m^2 * km / s * km / s
% = k * kg * km / s^2
% = MN

% convert MN to N
F = F * 1.0e+6; % [N]

== matlab function Environment&Dynamics/GPperturbation/MATLAB Function1 ==
  data: phi input double; lam input double; r input double; i input double; u input double; a output double; Re input double; GE input double; J2 input double
function a = fcn(phi, lam, r, i, u, Re, GE, J2)
%#codegen

% phi: latitude[rad]
% lam: longitude[rad]
% r  : distance from center of th earth to satellite[km]
% i  : inclination[rad]
% u  : w + th[rad]
% Re : radius of the earth[km]
% GE : geocentric gravitational constant[km^3/s^2]

% U20 = 3 * J2 * GE / 2 / r * (Re / r)^2 * (sin^2(phi) - 1 / 3)
% sin(phi) = sin(i) + sin(u)

r2 = r * r;
common = 3.0 * J2 * GE * Re * Re / r2 / r2;
% km^3 / s^2 * km * km / km^2 / km^2 = km / s^2

ci = cos(i);
si = sin(i);
cu = cos(u);
su = sin(u);

FR =  common / 2.0 * (3.0 * si * si * su * su - 1.0);
FS = -common * si * si * su * cu;
FW = -common * si * ci * su;

a = [FR; FS; FW]; % km / s^2

== matlab function Environment&Dynamics/Gravity Gradient/MATLAB Function ==
  data: R input double; T output double; GE input double; I input double
function T = fcn(R, GE, I)
%#codegen

% R: vector from center of the earth to satellite[km]
% GE : geocentric gravitational constant[km^3/s^2]
% I: inertia[kg m^2]

normR = norm(R);
R = R / normR;

T = 3.0 * GE / normR / normR / normR * cross(R, I * R);
% km^3 / s^2 / km / km / km * kg * m^2
% = kg * m^2 / s^2
% = N m

== matlab function Environment&Dynamics/OrbitalDynamics/orbital dynamics ==
  data: OE input double; th input double; r input double; F input double; d_OE output double; GE input double
function d_OE = diff_ele(OE,th,r,F,GE)
%#codegen
% calculate orbital elements update

a = OE(1);
e = OE(2);
i = OE(3);
ww = OE(5);

n = sqrt (GE / (a * a * a));
p = a * (1.0 -e * e);
h = sqrt(GE * p);

u = ww + th;

cu = cos(u);
ci = cos(i);
su = sin(u);
si = sin(i);
cth = cos(th);
sth = sin(th);

Fr = F(1);
Fs = F(2);
Fw = F(3);

da = 2.0 * a * a / h * (e * sth * Fr + p / r * Fs);
de = p / h * (sth * Fr + (cth + (e + cth) / (1.0 + e * cth)) * Fs);
di = r * cu / h * Fw;
dW = r * su / (h * si) * Fw;
if abs(e) > 1.0e-6
    d_w = - p / (e * h) * (cth * Fr - sth * (1.0 + r / p) * Fs) - dW * ci;
    dM =  n +1.0 / (n * a * a * e) * ((p * cth - 2.0 * e * r) * Fr - (p + r) * sth * Fs);
else
    d_w = -dW * ci;
    dM = n - 2.0 * r / n / a / a * Fr;
end

d_OE = [da,de,di,dW,d_w,dM];

== matlab function Environment&Dynamics/RigidBodyDynamics/dynamics ==
  data: q input double; rate input double; d_q output double; t_cont input double; t_dist input double; hw input double; d_rate output double; I input double
function [d_q, d_rate] = att_dyn(q, rate, t_cont, t_dist, hw, I)

%#codegen

% dq/dt = 1/2 * [    0      -rate'] * q
%               [ rate -rate_tilde] 
d_q = 0.5 * [       0 -rate(1) -rate(2) -rate(3);...
              rate(1)        0  rate(3) -rate(2);...
              rate(2) -rate(3)       0   rate(1);...
              rate(3)  rate(2) -rate(1)        0] * q;
     
rate_tilde=[       0 -rate(3)  rate(2); ...
             rate(3)        0 -rate(1); ...
            -rate(2)  rate(1)        0];

% I * d_rate + rate_tilde * (I * rate + hw) = t_cont + t_dist
d_rate = (I)\(t_cont + t_dist - rate_tilde * (I * rate + hw));

== matlab function Environment&Dynamics/SRP/SRP ==
  data: r input double; F output double; flag input double; pSR input double; CR input double; A input double
function F = fcn(r, flag, pSR, CR, A)
%#codegen

% r  : normalized vector from satellite to sun
% pSR: pressure of solar radiation[N/m^2]
% CR : reflectivity
% A  : cross section of satellite[m^2]

if flag == 1
    F = -pSR * CR * A * r;
    % N / m^2 * m^2 = N
else
    F = [0.0; 0.0; 0.0];
end

== matlab function GravityGradient/gravity_gradient ==
  data: ra input double; Tgg output double; I input double
function Tgg = g_g(ra,I)
%#codegen
% y = [xx xy xz;xy yy yz;xz yz zz];
GE=3.986004415*(10^5); % km^3/s^2
R=6378.1363; %km
Tgg=3.0*GE/(R*R*R)*...
    [ra(2)*ra(3)*(I(3,3)-I(2,2))+ra(3)*ra(1)*I(1,2)-ra(1)*ra(2)*I(1,3)+(ra(3)*ra(3)-ra(2)*ra(2))*I(2,3);...
    ra(3)*ra(1)*(I(1,1)-I(3,3))+ra(1)*ra(2)*I(1,2)-ra(2)*ra(3)*I(1,2)+(ra(1)*ra(1)-ra(3)*ra(3))*I(1,3);...
    ra(1)*ra(2)*(I(2,2)-I(1,1))+ra(2)*ra(3)*I(1,2)-ra(3)*ra(1)*I(2,3)+(ra(2)*ra(2)-ra(1)*ra(1))*I(1,2)];

== matlab function GravityGradient/radius_vec ==
  data: q input double; ra_vec output double
function ra_vec = radius(q)
%#codegen

ra_vec=[	q(1)*q(1)- q(2)*q(2)- q(3)*q(3)+ q(4)*q(4);...			
		2.0 * (q(1)* q(2)- q(3)*q(4));...						
		2.0 * (q(1)* q(3)+ q(2)*q(4))];
